simulink model "zad_4_sch_wyprzedzajace"  (R2022b)
settings: Solver=FixedStepAuto  StartTime=0.0  StopTime=10.0  FixedStep=0.0001  RelTol=1e-3
values from neighbouring files (symbols this model uses):
  a21 = 1/(2*m)*x30^2*FemP1/FemP2^2*exp(-x10/FemP2)    [zad_4.m]
  a23 = -1/(m)*x30*FemP1/FemP2*exp(-x10/FemP2)    [zad_4.m]
  a31 = 1/f1*exp(x10/f2)*(ki*u10+ci-x30)    [zad_4.m]
  a33 = -f2/f1*exp(x10/f2)    [zad_4.m]
  b31 = ki*f2/f1*exp(x10/f2)    [zad_4.m]
  g = 9.81    [zad_4.m]
  k = -acker(A, B(:,1), -s)    [zad_4.m]
  xd = d-bd    (= 0.0192)    [zad_4.m]
settings Model: Creator=MPatr  LastModifiedBy=MPatr

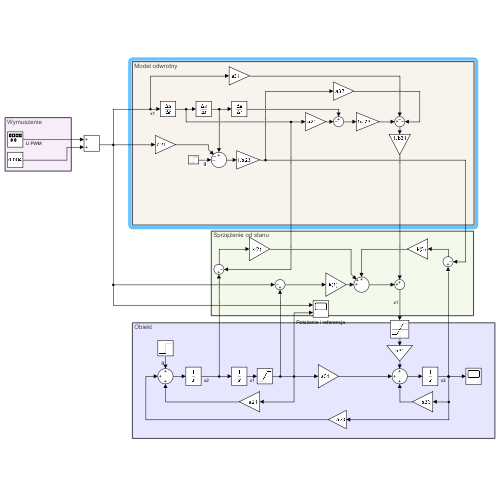
[thumbnail: Simulink's stored preview of the top-level diagram]
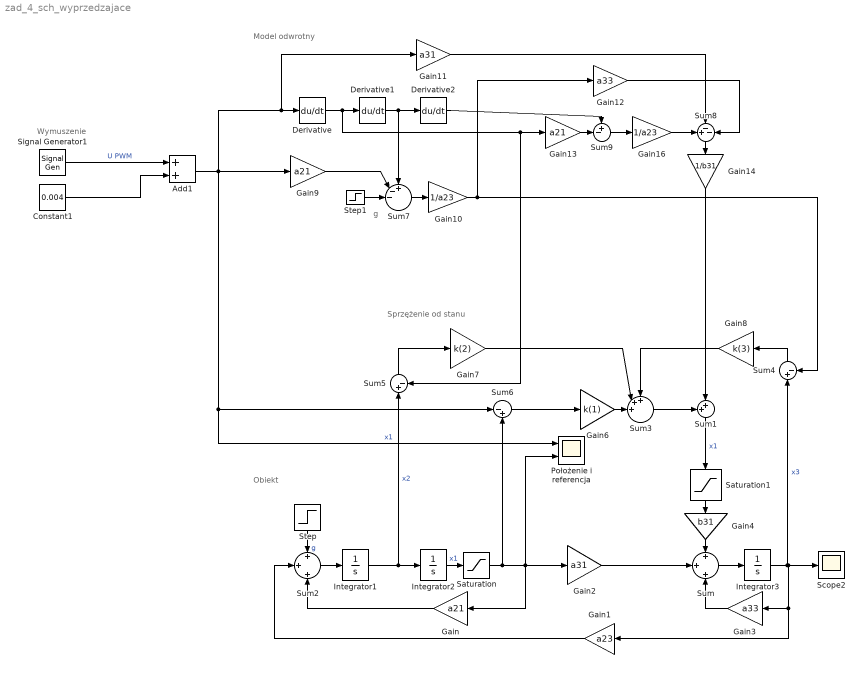
== system zad_4_sch_wyprzedzajace ==
  note: g
  note: Sprzężenie od stanu
  note: Model odwrotny
  note: Obiekt
  note: Wymuszenie
  Add1 : Sum
  Constant1 : Constant  Value=0.004
  Derivative : Derivative
  Derivative1 : Derivative
  Derivative2 : Derivative
  Gain : Gain  Gain=a21
  Gain1 : Gain  Gain=a23
  Gain10 : Gain  Gain=1/a23
  Gain11 : Gain  Gain=a31
  Gain12 : Gain  Gain=a33
  Gain13 : Gain  Gain=a21
  Gain14 : Gain  Gain=1/b31
  Gain16 : Gain  Gain=1/a23
  Gain2 : Gain  Gain=a31
  Gain3 : Gain  Gain=a33
  Gain4 : Gain  Gain=b31
  Gain6 : Gain  Gain=k(1)
  Gain7 : Gain  Gain=k(2)
  Gain8 : Gain  Gain=k(3)
  Gain9 : Gain  Gain=a21
  Integrator1 : Integrator
  Integrator2 : Integrator  InitialCondition=xd
  Integrator3 : Integrator
  Położenie i referencja : Scope  NumInputPorts=2
  Saturation : Saturate  UpperLimit=xd  LowerLimit=0
  Saturation1 : Saturate  UpperLimit=1  LowerLimit=0
  Scope2 : Scope
  Signal Generator1 : SignalGenerator  Amplitude=.002  Frequency=8  Units=rad/sec
  Step : Step  Time=0  After=g  SampleTime=0
  Step1 : Step  Time=0  After=g  SampleTime=0
  Sum : Sum  Inputs=+|+|+
  Sum1 : Sum  Inputs=++|
  Sum2 : Sum  Inputs=+|+|+
  Sum3 : Sum  Inputs=+++||
  Sum4 : Sum  Inputs=|+-
  Sum5 : Sum  Inputs=|+-
  Sum6 : Sum  Inputs=|-+
  Sum7 : Sum  Inputs=+--||
  Sum8 : Sum  Inputs=+--
  Sum9 : Sum  Inputs=+-|
  wires:
  Sum1/1 -> Saturation1/1  "x1"
  Gain7/1 -> Sum3/2
  Sum6/1 -> Gain6/1
  Constant1/1 -> Add1/2
  Sum/1 -> Integrator3/1
  Add1/1 -> Położenie i referencja/1, Sum6/1, Gain9/1, Gain11/1, Derivative/1  "x1"
  Gain1/1 -> Sum2/2
  Gain2/1 -> Sum/2
  Gain6/1 -> Sum3/3
  Sum4/1 -> Gain8/1
  Integrator1/1 -> Integrator2/1, Sum5/1  "x2"
  Sum3/1 -> Sum1/1
  Signal Generator1/1 -> Add1/1  "U PWM"
  Gain8/1 -> Sum3/1
  Gain/1 -> Sum2/3
  Gain3/1 -> Sum/3
  Sum5/1 -> Gain7/1
  Integrator2/1 -> Saturation/1  "x1"
  Step/1 -> Sum2/1  "g"
  Gain4/1 -> Sum/1
  Integrator3/1 -> Gain1/1, Gain3/1, Scope2/1, Sum4/1  "x3"
  Sum2/1 -> Integrator1/1
  Derivative/1 -> Derivative1/1, Sum5/2, Gain13/1
  Derivative1/1 -> Derivative2/1, Sum7/1
  Step1/1 -> Sum7/3
  Gain9/1 -> Sum7/2
  Sum7/1 -> Gain10/1
  Gain10/1 -> Gain12/1, Sum4/2
  Sum8/1 -> Gain14/1
  Gain11/1 -> Sum8/2
  Gain12/1 -> Sum8/3
  Derivative2/1 -> Sum9/1
  Sum9/1 -> Gain16/1
  Gain14/1 -> Sum1/2
  Gain16/1 -> Sum8/1
  Saturation/1 -> Gain2/1, Położenie i referencja/2, Gain/1, Sum6/2
  Saturation1/1 -> Gain4/1
  Gain13/1 -> Sum9/2
